simulink model "dog_test"  (R2015a)
settings: Solver=ode45  StartTime=0.0  StopTime=11796  RelTol=1e-3
InitFcn:
  | %% DSPBuilder Start
  | alt_dspbuilder_update_model(bdroot)
  | %% DSPBuilder End
libraries: allblocks_alteradspbuilder2 x539
(part 5 of 6)

== system dog_test/Gaussian_scale4/Subsystem ==
  valid_in : Inport
  eof_in : Inport  Port=2
  Comparator : allblocks_alteradspbuilder2/Comparator  direction=a == b  pipeline_display=0  allowFloatingPointOverride=on  logOutputs=off  logFile=C:\Users\ASUS\Desktop\sift_fpga_final\Gaussian filter 5x5\tb_dog_test\dog%5Ftest_Gaussian%5Fscale4_Subsystem_Comparator.fixedpointlog
  Comparator1 : allblocks_alteradspbuilder2/Comparator  direction=a < b  pipeline_display=0  allowFloatingPointOverride=on  logOutputs=off  logFile=C:\Users\ASUS\Desktop\sift_fpga_final\Gaussian filter 5x5\tb_dog_test\dog%5Ftest_Gaussian%5Fscale4_Subsystem_Comparator1.fixedpointlog
  Comparator2 : allblocks_alteradspbuilder2/Comparator  direction=a > b  pipeline_display=0  allowFloatingPointOverride=on  logOutputs=off  logFile=C:\Users\ASUS\Desktop\sift_fpga_final\Gaussian filter 5x5\tb_dog_test\dog%5Ftest_Gaussian%5Fscale4_Subsystem_Comparator2.fixedpointlog
  Comparator3 : allblocks_alteradspbuilder2/Comparator  direction=a > b  pipeline_display=0  allowFloatingPointOverride=on  logOutputs=off  logFile=C:\Users\ASUS\Desktop\sift_fpga_final\Gaussian filter 5x5\tb_dog_test\dog%5Ftest_Gaussian%5Fscale4_Subsystem_Comparator3.fixedpointlog
  Comparator4 : allblocks_alteradspbuilder2/Comparator  direction=a > b  pipeline_display=0  allowFloatingPointOverride=on  logOutputs=off  logFile=C:\Users\ASUS\Desktop\sift_fpga_final\Gaussian filter 5x5\tb_dog_test\dog%5Ftest_Gaussian%5Fscale4_Subsystem_Comparator4.fixedpointlog
  Comparator5 : allblocks_alteradspbuilder2/Comparator  direction=a > b  pipeline_display=0  allowFloatingPointOverride=on  logOutputs=off  logFile=C:\Users\ASUS\Desktop\sift_fpga_final\Gaussian filter 5x5\tb_dog_test\dog%5Ftest_Gaussian%5Fscale4_Subsystem_Comparator5.fixedpointlog
  Comparator6 : allblocks_alteradspbuilder2/Comparator  direction=a == b  pipeline_display=0  allowFloatingPointOverride=on  logOutputs=off  logFile=C:\Users\ASUS\Desktop\sift_fpga_final\Gaussian filter 5x5\tb_dog_test\dog%5Ftest_Gaussian%5Fscale4_Subsystem_Comparator6.fixedpointlog
  Comparator7 : allblocks_alteradspbuilder2/Comparator  direction=a == b  pipeline_display=0  allowFloatingPointOverride=on  logOutputs=off  logFile=C:\Users\ASUS\Desktop\sift_fpga_final\Gaussian filter 5x5\tb_dog_test\dog%5Ftest_Gaussian%5Fscale4_Subsystem_Comparator7.fixedpointlog
  Comparator8 : allblocks_alteradspbuilder2/Comparator  direction=a == b  pipeline_display=0  allowFloatingPointOverride=on  logOutputs=off  logFile=C:\Users\ASUS\Desktop\sift_fpga_final\Gaussian filter 5x5\tb_dog_test\dog%5Ftest_Gaussian%5Fscale4_Subsystem_Comparator8.fixedpointlog
  Constant : allblocks_alteradspbuilder2/Constant  mask_cst=643  BusType=Unsigned Integer  bwl=10  bwr=0  roundMode=Truncate  satMode=Wrap  SpecifyClock=off  allowFloatingPointOverride=on  logOutputs=off  logFile=C:\Users\ASUS\Desktop\sift_fpga_final\Gaussian filter 5x5\tb_dog_test\dog%5Ftest_Gaussian%5Fscale4_Subsystem_Constant.fixedpointlog
  Constant1 : allblocks_alteradspbuilder2/Constant  mask_cst=23  BusType=Unsigned Integer  bwl=10  bwr=0  roundMode=Truncate  satMode=Wrap  SpecifyClock=off  allowFloatingPointOverride=on  logOutputs=off  logFile=C:\Users\ASUS\Desktop\sift_fpga_final\Gaussian filter 5x5\tb_dog_test\dog%5Ftest_Gaussian%5Fscale4_Subsystem_Constant1.fixedpointlog
  Constant2 : allblocks_alteradspbuilder2/Constant  mask_cst=4  BusType=Unsigned Integer  bwl=10  bwr=0  roundMode=Truncate  satMode=Wrap  SpecifyClock=off  allowFloatingPointOverride=on  logOutputs=off  logFile=C:\Users\ASUS\Desktop\sift_fpga_final\Gaussian filter 5x5\tb_dog_test\dog%5Ftest_Gaussian%5Fscale4_Subsystem_Constant2.fixedpointlog
  Constant3 : allblocks_alteradspbuilder2/Constant  mask_cst=26  BusType=Unsigned Integer  bwl=10  bwr=0  roundMode=Truncate  satMode=Wrap  SpecifyClock=off  allowFloatingPointOverride=on  logOutputs=off  logFile=C:\Users\ASUS\Desktop\sift_fpga_final\Gaussian filter 5x5\tb_dog_test\dog%5Ftest_Gaussian%5Fscale4_Subsystem_Constant3.fixedpointlog
  Constant4 : allblocks_alteradspbuilder2/Constant  mask_cst=3  BusType=Unsigned Integer  bwl=10  bwr=0  roundMode=Truncate  satMode=Wrap  SpecifyClock=off  allowFloatingPointOverride=on  logOutputs=off  logFile=C:\Users\ASUS\Desktop\sift_fpga_final\Gaussian filter 5x5\tb_dog_test\dog%5Ftest_Gaussian%5Fscale4_Subsystem_Constant4.fixedpointlog
  Constant5 : allblocks_alteradspbuilder2/Constant  mask_cst=0  BusType=Unsigned Integer  bwl=10  bwr=0  roundMode=Truncate  satMode=Wrap  SpecifyClock=off  allowFloatingPointOverride=on  logOutputs=off  logFile=C:\Users\ASUS\Desktop\sift_fpga_final\Gaussian filter 5x5\tb_dog_test\dog%5Ftest_Gaussian%5Fscale4_Subsystem_Constant5.fixedpointlog
  Constant6 : allblocks_alteradspbuilder2/Constant  mask_cst=23  BusType=Unsigned Integer  bwl=10  bwr=0  roundMode=Truncate  satMode=Wrap  SpecifyClock=off  allowFloatingPointOverride=on  logOutputs=off  logFile=C:\Users\ASUS\Desktop\sift_fpga_final\Gaussian filter 5x5\tb_dog_test\dog%5Ftest_Gaussian%5Fscale4_Subsystem_Constant6.fixedpointlog
  Constant7 : allblocks_alteradspbuilder2/Constant  mask_cst=4  BusType=Unsigned Integer  bwl=10  bwr=0  roundMode=Truncate  satMode=Wrap  SpecifyClock=off  allowFloatingPointOverride=on  logOutputs=off  logFile=C:\Users\ASUS\Desktop\sift_fpga_final\Gaussian filter 5x5\tb_dog_test\dog%5Ftest_Gaussian%5Fscale4_Subsystem_Constant7.fixedpointlog
  Constant8 : allblocks_alteradspbuilder2/Constant  mask_cst=27  BusType=Unsigned Integer  bwl=10  bwr=0  roundMode=Truncate  satMode=Wrap  SpecifyClock=off  allowFloatingPointOverride=on  logOutputs=off  logFile=C:\Users\ASUS\Desktop\sift_fpga_final\Gaussian filter 5x5\tb_dog_test\dog%5Ftest_Gaussian%5Fscale4_Subsystem_Constant8.fixedpointlog
  Counter : allblocks_alteradspbuilder2/Counter  BusType=Unsigned Integer  bwl=10  bwr=0  use_modulo=on  modulo=644  SpecifyClock=off  direction=Increment  use_sload=off  use_sset=off  svalue=1  use_clk_ena=off  use_ena=on  use_sclr=on  pipeline_display=1
  Counter1 : allblocks_alteradspbuilder2/Counter  BusType=Unsigned Integer  bwl=10  bwr=0  use_modulo=on  modulo=484  SpecifyClock=off  direction=Increment  use_sload=off  use_sset=off  svalue=1  use_clk_ena=off  use_ena=on  use_sclr=on  pipeline_display=1
  Counter2 : allblocks_alteradspbuilder2/Counter  BusType=Unsigned Integer  bwl=5  bwr=0  use_modulo=on  modulo=24  SpecifyClock=off  direction=Increment  use_sload=off  use_sset=on  svalue=1  use_clk_ena=off  use_ena=on  use_sclr=off  pipeline_display=1
  Logical Bit Operator{,1..3,5..6} (6 alike) : allblocks_alteradspbuilder2/Logical Bit Operator  LogicalOperator=AND  user_inputs=2  pipeline_display=0
  Logical Bit Operator4 : allblocks_alteradspbuilder2/Logical Bit Operator  LogicalOperator=OR  user_inputs=3  pipeline_display=0
  Logical Bit Operator7 : allblocks_alteradspbuilder2/Logical Bit Operator  LogicalOperator=AND  user_inputs=3  pipeline_display=0
  valid_out : Outport
  sof_out : Outport  Port=2
  eof_out : Outport  Port=3
  wires:
  Logical Bit Operator3/1 -> Logical Bit Operator4/2
  Counter2/1 -> [counter_eof]
  [valid_in] -> Logical Bit Operator1/1
  Constant1/1 -> Comparator1/2
  Constant2/1 -> Comparator2/2
  Constant3/1 -> Comparator3/2
  Logical Bit Operator4/1 -> Logical Bit Operator1/2
  [valid_in] -> Logical Bit Operator5/1
  Comparator/1 -> Logical Bit Operator/2
  [counter_col] -> Comparator3/1
  [counter_eof] -> Comparator5/1
  [counter_col] -> Comparator/1
  Constant5/1 -> Comparator5/2
  eof_in/1 -> [eof_in]
  [eof_in] -> Counter1/2
  Logical Bit Operator1/1 -> [valid_out]
  Constant/1 -> Comparator/2
  Logical Bit Operator/1 -> Counter1/1
  Comparator2/1 -> Logical Bit Operator2/2
  Comparator3/1 -> Logical Bit Operator3/1
  Comparator4/1 -> Logical Bit Operator3/2
  Logical Bit Operator2/1 -> Logical Bit Operator4/1
  valid_in/1 -> [valid_in]
  [eof_in] -> Counter/2
  Counter1/1 -> [counter_row]
  [counter_row] -> Comparator2/1
  [counter_row] -> Comparator4/1
  Constant4/1 -> Comparator4/2
  [valid_in] -> Logical Bit Operator/1, Counter/1
  Counter/1 -> [counter_col]
  [counter_col] -> Comparator1/1
  Comparator1/1 -> Logical Bit Operator2/1
  Comparator7/1 -> Logical Bit Operator7/2
  [valid_in] -> Logical Bit Operator7/1
  Constant6/1 -> Comparator6/2
  [sof_out] -> sof_out/1
  [counter_row] -> Comparator7/1
  Comparator8/1 -> Logical Bit Operator7/3
  [counter_col] -> Comparator8/1
  [valid_in] -> Logical Bit Operator6/1
  [eof_out] -> eof_out/1
  Logical Bit Operator7/1 -> [sof_out]
  [valid_out] -> valid_out/1
  [counter_eof] -> Comparator6/1
  Constant8/1 -> Comparator8/2
  Comparator6/1 -> Logical Bit Operator6/2
  Comparator5/1 -> Logical Bit Operator5/2, Logical Bit Operator4/3
  Logical Bit Operator6/1 -> [eof_out]
  Constant7/1 -> Comparator7/2
  [eof_in] -> Counter2/1
  Logical Bit Operator5/1 -> Counter2/2

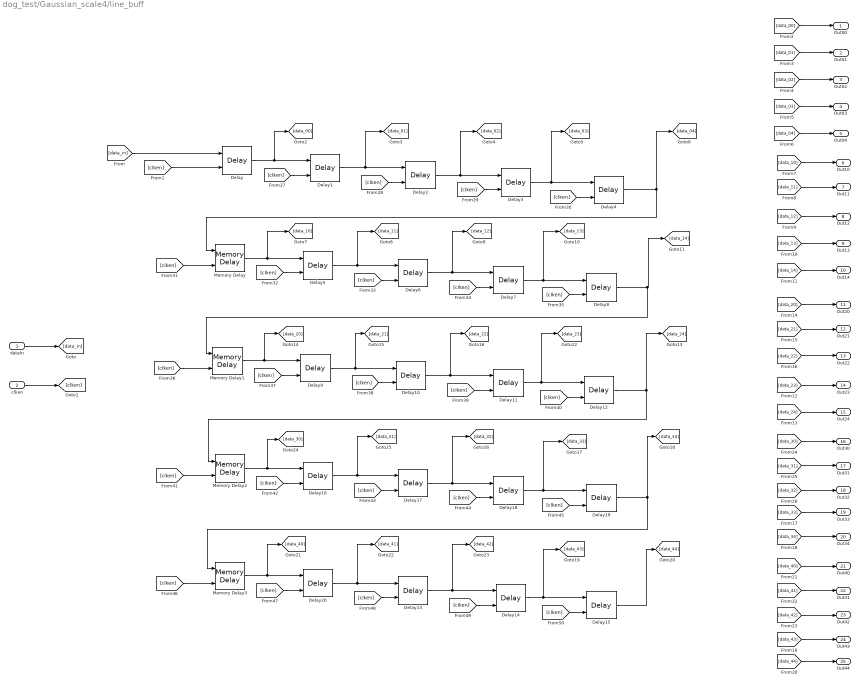
== system dog_test/Gaussian_scale4/line_buff ==
  dataIn : Inport
  clken : Inport  Port=2
  Delay : allblocks_alteradspbuilder2/Delay  pipeline=1  pipeline_display=1  ClockPhase=1  use_ena=on  use_sclr=off  allowFloatingPointOverride=on  logOutputs=off  logFile=C:\Users\ASUS\Desktop\sift_fpga_final\Gaussian filter 5x5\tb_dog_test\dog%5Ftest_Gaussian%5Fscale4_line%5Fbuff_Delay.fixedpointlog  use_init=off  reset_value=1
  Delay1 : allblocks_alteradspbuilder2/Delay  pipeline=1  pipeline_display=1  ClockPhase=1  use_ena=on  use_sclr=off  allowFloatingPointOverride=on  logOutputs=off  logFile=C:\Users\ASUS\Desktop\sift_fpga_final\Gaussian filter 5x5\tb_dog_test\dog%5Ftest_Gaussian%5Fscale4_line%5Fbuff_Delay1.fixedpointlog  use_init=off  reset_value=1
  Delay10 : allblocks_alteradspbuilder2/Delay  pipeline=1  pipeline_display=1  ClockPhase=1  use_ena=on  use_sclr=off  allowFloatingPointOverride=on  logOutputs=off  logFile=C:\Users\ASUS\Desktop\sift_fpga_final\Gaussian filter 5x5\tb_dog_test\dog%5Ftest_Gaussian%5Fscale4_line%5Fbuff_Delay10.fixedpointlog  use_init=off  reset_value=1
  Delay11 : allblocks_alteradspbuilder2/Delay  pipeline=1  pipeline_display=1  ClockPhase=1  use_ena=on  use_sclr=off  allowFloatingPointOverride=on  logOutputs=off  logFile=C:\Users\ASUS\Desktop\sift_fpga_final\Gaussian filter 5x5\tb_dog_test\dog%5Ftest_Gaussian%5Fscale4_line%5Fbuff_Delay11.fixedpointlog  use_init=off  reset_value=1
  Delay12 : allblocks_alteradspbuilder2/Delay  pipeline=1  pipeline_display=1  ClockPhase=1  use_ena=on  use_sclr=off  allowFloatingPointOverride=on  logOutputs=off  logFile=C:\Users\ASUS\Desktop\sift_fpga_final\Gaussian filter 5x5\tb_dog_test\dog%5Ftest_Gaussian%5Fscale4_line%5Fbuff_Delay12.fixedpointlog  use_init=off  reset_value=1
  Delay13 : allblocks_alteradspbuilder2/Delay  pipeline=1  pipeline_display=1  ClockPhase=1  use_ena=on  use_sclr=off  allowFloatingPointOverride=on  logOutputs=off  logFile=C:\Users\ASUS\Desktop\sift_fpga_final\Gaussian filter 5x5\tb_dog_test\dog%5Ftest_Gaussian%5Fscale4_line%5Fbuff_Delay13.fixedpointlog  use_init=off  reset_value=1
  Delay14 : allblocks_alteradspbuilder2/Delay  pipeline=1  pipeline_display=1  ClockPhase=1  use_ena=on  use_sclr=off  allowFloatingPointOverride=on  logOutputs=off  logFile=C:\Users\ASUS\Desktop\sift_fpga_final\Gaussian filter 5x5\tb_dog_test\dog%5Ftest_Gaussian%5Fscale4_line%5Fbuff_Delay14.fixedpointlog  use_init=off  reset_value=1
  Delay15 : allblocks_alteradspbuilder2/Delay  pipeline=1  pipeline_display=1  ClockPhase=1  use_ena=on  use_sclr=off  allowFloatingPointOverride=on  logOutputs=off  logFile=C:\Users\ASUS\Desktop\sift_fpga_final\Gaussian filter 5x5\tb_dog_test\dog%5Ftest_Gaussian%5Fscale4_line%5Fbuff_Delay15.fixedpointlog  use_init=off  reset_value=1
  Delay16 : allblocks_alteradspbuilder2/Delay  pipeline=1  pipeline_display=1  ClockPhase=1  use_ena=on  use_sclr=off  allowFloatingPointOverride=on  logOutputs=off  logFile=C:\Users\ASUS\Desktop\sift_fpga_final\Gaussian filter 5x5\tb_dog_test\dog%5Ftest_Gaussian%5Fscale4_line%5Fbuff_Delay16.fixedpointlog  use_init=off  reset_value=1
  Delay17 : allblocks_alteradspbuilder2/Delay  pipeline=1  pipeline_display=1  ClockPhase=1  use_ena=on  use_sclr=off  allowFloatingPointOverride=on  logOutputs=off  logFile=C:\Users\ASUS\Desktop\sift_fpga_final\Gaussian filter 5x5\tb_dog_test\dog%5Ftest_Gaussian%5Fscale4_line%5Fbuff_Delay17.fixedpointlog  use_init=off  reset_value=1
  Delay18 : allblocks_alteradspbuilder2/Delay  pipeline=1  pipeline_display=1  ClockPhase=1  use_ena=on  use_sclr=off  allowFloatingPointOverride=on  logOutputs=off  logFile=C:\Users\ASUS\Desktop\sift_fpga_final\Gaussian filter 5x5\tb_dog_test\dog%5Ftest_Gaussian%5Fscale4_line%5Fbuff_Delay18.fixedpointlog  use_init=off  reset_value=1
  Delay19 : allblocks_alteradspbuilder2/Delay  pipeline=1  pipeline_display=1  ClockPhase=1  use_ena=on  use_sclr=off  allowFloatingPointOverride=on  logOutputs=off  logFile=C:\Users\ASUS\Desktop\sift_fpga_final\Gaussian filter 5x5\tb_dog_test\dog%5Ftest_Gaussian%5Fscale4_line%5Fbuff_Delay19.fixedpointlog  use_init=off  reset_value=1
  Delay2 : allblocks_alteradspbuilder2/Delay  pipeline=1  pipeline_display=1  ClockPhase=1  use_ena=on  use_sclr=off  allowFloatingPointOverride=on  logOutputs=off  logFile=C:\Users\ASUS\Desktop\sift_fpga_final\Gaussian filter 5x5\tb_dog_test\dog%5Ftest_Gaussian%5Fscale4_line%5Fbuff_Delay2.fixedpointlog  use_init=off  reset_value=1
  Delay20 : allblocks_alteradspbuilder2/Delay  pipeline=1  pipeline_display=1  ClockPhase=1  use_ena=on  use_sclr=off  allowFloatingPointOverride=on  logOutputs=off  logFile=C:\Users\ASUS\Desktop\sift_fpga_final\Gaussian filter 5x5\tb_dog_test\dog%5Ftest_Gaussian%5Fscale4_line%5Fbuff_Delay20.fixedpointlog  use_init=off  reset_value=1
  Delay3 : allblocks_alteradspbuilder2/Delay  pipeline=1  pipeline_display=1  ClockPhase=1  use_ena=on  use_sclr=off  allowFloatingPointOverride=on  logOutputs=off  logFile=C:\Users\ASUS\Desktop\sift_fpga_final\Gaussian filter 5x5\tb_dog_test\dog%5Ftest_Gaussian%5Fscale4_line%5Fbuff_Delay3.fixedpointlog  use_init=off  reset_value=1
  Delay4 : allblocks_alteradspbuilder2/Delay  pipeline=1  pipeline_display=1  ClockPhase=1  use_ena=on  use_sclr=off  allowFloatingPointOverride=on  logOutputs=off  logFile=C:\Users\ASUS\Desktop\sift_fpga_final\Gaussian filter 5x5\tb_dog_test\dog%5Ftest_Gaussian%5Fscale4_line%5Fbuff_Delay4.fixedpointlog  use_init=off  reset_value=1
  Delay5 : allblocks_alteradspbuilder2/Delay  pipeline=1  pipeline_display=1  ClockPhase=1  use_ena=on  use_sclr=off  allowFloatingPointOverride=on  logOutputs=off  logFile=C:\Users\ASUS\Desktop\sift_fpga_final\Gaussian filter 5x5\tb_dog_test\dog%5Ftest_Gaussian%5Fscale4_line%5Fbuff_Delay5.fixedpointlog  use_init=off  reset_value=1
  Delay6 : allblocks_alteradspbuilder2/Delay  pipeline=1  pipeline_display=1  ClockPhase=1  use_ena=on  use_sclr=off  allowFloatingPointOverride=on  logOutputs=off  logFile=C:\Users\ASUS\Desktop\sift_fpga_final\Gaussian filter 5x5\tb_dog_test\dog%5Ftest_Gaussian%5Fscale4_line%5Fbuff_Delay6.fixedpointlog  use_init=off  reset_value=1
  Delay7 : allblocks_alteradspbuilder2/Delay  pipeline=1  pipeline_display=1  ClockPhase=1  use_ena=on  use_sclr=off  allowFloatingPointOverride=on  logOutputs=off  logFile=C:\Users\ASUS\Desktop\sift_fpga_final\Gaussian filter 5x5\tb_dog_test\dog%5Ftest_Gaussian%5Fscale4_line%5Fbuff_Delay7.fixedpointlog  use_init=off  reset_value=1
  Delay8 : allblocks_alteradspbuilder2/Delay  pipeline=1  pipeline_display=1  ClockPhase=1  use_ena=on  use_sclr=off  allowFloatingPointOverride=on  logOutputs=off  logFile=C:\Users\ASUS\Desktop\sift_fpga_final\Gaussian filter 5x5\tb_dog_test\dog%5Ftest_Gaussian%5Fscale4_line%5Fbuff_Delay8.fixedpointlog  use_init=off  reset_value=1
  Delay9 : allblocks_alteradspbuilder2/Delay  pipeline=1  pipeline_display=1  ClockPhase=1  use_ena=on  use_sclr=off  allowFloatingPointOverride=on  logOutputs=off  logFile=C:\Users\ASUS\Desktop\sift_fpga_final\Gaussian filter 5x5\tb_dog_test\dog%5Ftest_Gaussian%5Fscale4_line%5Fbuff_Delay9.fixedpointlog  use_init=off  reset_value=1
  Memory Delay : allblocks_alteradspbuilder2/Memory Delay  BusType=Unsigned Integer  bwl=8  bwr=0  pipeline=640  pipeline_display=640  ram_type=AUTO  use_ena=on  use_sclr=off  allowFloatingPointOverride=on  logOutputs=off  logFile=C:\Users\ASUS\Desktop\sift_fpga_final\Gaussian filter 5x5\tb_dog_test\dog%5Ftest_Gaussian%5Fscale4_line%5Fbuff_Memory+Delay.fixedpointlog
  Memory Delay1 : allblocks_alteradspbuilder2/Memory Delay  BusType=Unsigned Integer  bwl=8  bwr=0  pipeline=640  pipeline_display=640  ram_type=AUTO  use_ena=on  use_sclr=off  allowFloatingPointOverride=on  logOutputs=off  logFile=C:\Users\ASUS\Desktop\sift_fpga_final\Gaussian filter 5x5\tb_dog_test\dog%5Ftest_Gaussian%5Fscale4_line%5Fbuff_Memory+Delay1.fixedpointlog
  Memory Delay2 : allblocks_alteradspbuilder2/Memory Delay  BusType=Unsigned Integer  bwl=8  bwr=0  pipeline=640  pipeline_display=640  ram_type=AUTO  use_ena=on  use_sclr=off  allowFloatingPointOverride=on  logOutputs=off  logFile=C:\Users\ASUS\Desktop\sift_fpga_final\Gaussian filter 5x5\tb_dog_test\dog%5Ftest_Gaussian%5Fscale4_line%5Fbuff_Memory+Delay2.fixedpointlog
  Memory Delay3 : allblocks_alteradspbuilder2/Memory Delay  BusType=Unsigned Integer  bwl=8  bwr=0  pipeline=640  pipeline_display=640  ram_type=AUTO  use_ena=on  use_sclr=off  allowFloatingPointOverride=on  logOutputs=off  logFile=C:\Users\ASUS\Desktop\sift_fpga_final\Gaussian filter 5x5\tb_dog_test\dog%5Ftest_Gaussian%5Fscale4_line%5Fbuff_Memory+Delay3.fixedpointlog
  Out00 : Outport
  Out01 : Outport  Port=2
  Out02 : Outport  Port=3
  Out03 : Outport  Port=4
  Out04 : Outport  Port=5
  Out10 : Outport  Port=6
  Out11 : Outport  Port=7
  Out12 : Outport  Port=8
  Out13 : Outport  Port=9
  Out14 : Outport  Port=10
  Out20 : Outport  Port=11
  Out21 : Outport  Port=12
  Out22 : Outport  Port=13
  Out23 : Outport  Port=14
  Out24 : Outport  Port=15
  Out30 : Outport  Port=16
  Out31 : Outport  Port=17
  Out32 : Outport  Port=18
  Out33 : Outport  Port=19
  Out34 : Outport  Port=20
  Out40 : Outport  Port=21
  Out41 : Outport  Port=22
  Out42 : Outport  Port=23
  Out43 : Outport  Port=24
  Out44 : Outport  Port=25
  wires:
  [clken] -> Delay9/2
  [data_04] -> Out04/1
  [data_02] -> Out02/1
  [clken] -> Memory Delay1/2
  [data_44] -> Out44/1
  [data_33] -> Out33/1
  [clken] -> Delay4/2
  [clken] -> Delay11/2
  [data_32] -> Out32/1
  [data_31] -> Out31/1
  [data_40] -> Out40/1
  [data_43] -> Out43/1
  [data_42] -> Out42/1
  Delay11/1 -> [data_23], Delay12/1
  Memory Delay1/1 -> [data_20], Delay9/1
  [data_41] -> Out41/1
  Delay9/1 -> [data_21], Delay10/1
  [clken] -> Delay12/2
  [data_34] -> Out34/1
  [data_30] -> Out30/1
  Delay/1 -> [data_00], Delay1/1
  [clken] -> Delay1/2
  [clken] -> Delay/2
  [data_03] -> Out03/1
  [clken] -> Delay10/2
  Delay8/1 -> Memory Delay1/1, [data_14]
  Delay10/1 -> [data_22], Delay11/1
  [data_12] -> Out12/1
  dataIn/1 -> [data_in]
  Memory Delay3/1 -> [data_40], Delay20/1
  [clken] -> Memory Delay/2
  [clken] -> Delay2/2
  [data_22] -> Out22/1
  [clken] -> Delay14/2
  Delay17/1 -> [data_32], Delay18/1
  [clken] -> Delay20/2
  [data_10] -> Out10/1
  [data_21] -> Out21/1
  Delay12/1 -> [data_24], Memory Delay2/1
  Delay4/1 -> Memory Delay/1, [data_04]
  [clken] -> Delay3/2
  Delay2/1 -> [data_02], Delay3/1
  [clken] -> Memory Delay2/2
  [data_23] -> Out23/1
  [data_13] -> Out13/1
  clken/1 -> [clken]
  [data_11] -> Out11/1
  Delay18/1 -> [data_33], Delay19/1
  [data_20] -> Out20/1
  Delay1/1 -> [data_01], Delay2/1
  [data_24] -> Out24/1
  Memory Delay2/1 -> [data_30], Delay16/1
  [clken] -> Delay16/2
  [data_14] -> Out14/1
  [data_00] -> Out00/1
  [clken] -> Delay15/2
  [clken] -> Memory Delay3/2
  [data_01] -> Out01/1
  [data_in] -> Delay/1
  [clken] -> Delay7/2
  Delay19/1 -> Memory Delay3/1, [data_34]
  Delay14/1 -> [data_43], Delay15/1
  Memory Delay/1 -> [data_10], Delay5/1
  Delay5/1 -> [data_11], Delay6/1
  Delay16/1 -> [data_31], Delay17/1
  [clken] -> Delay6/2
  Delay6/1 -> [data_12], Delay7/1
  [clken] -> Delay13/2
  Delay3/1 -> [data_03], Delay4/1
  Delay15/1 -> [data_44]
  [clken] -> Delay18/2
  Delay13/1 -> [data_42], Delay14/1
  [clken] -> Delay5/2
  Delay7/1 -> [data_13], Delay8/1
  Delay20/1 -> [data_41], Delay13/1
  [clken] -> Delay17/2
  [clken] -> Delay19/2
  [clken] -> Delay8/2

== system dog_test/calculate_key_point/Subsystem ==
  dataIn : Inport
  clken : Inport  Port=2
  Delay : allblocks_alteradspbuilder2/Delay  pipeline=1  pipeline_display=1  ClockPhase=1  use_ena=on  use_sclr=off  allowFloatingPointOverride=on  logOutputs=off  logFile=C:\Users\ASUS\Desktop\sift_fpga_final\Gaussian filter 5x5\tb_dog_test\dog%5Ftest_calculate%5Fkey%5Fpoint_Subsystem_Delay.fixedpointlog  use_init=off  reset_value=1
  Delay1 : allblocks_alteradspbuilder2/Delay  pipeline=1  pipeline_display=1  ClockPhase=1  use_ena=on  use_sclr=off  allowFloatingPointOverride=on  logOutputs=off  logFile=C:\Users\ASUS\Desktop\sift_fpga_final\Gaussian filter 5x5\tb_dog_test\dog%5Ftest_calculate%5Fkey%5Fpoint_Subsystem_Delay1.fixedpointlog  use_init=off  reset_value=1
  Delay10 : allblocks_alteradspbuilder2/Delay  pipeline=1  pipeline_display=1  ClockPhase=1  use_ena=on  use_sclr=off  allowFloatingPointOverride=on  logOutputs=off  logFile=C:\Users\ASUS\Desktop\sift_fpga_final\Gaussian filter 5x5\tb_dog_test\dog%5Ftest_calculate%5Fkey%5Fpoint_Subsystem_Delay10.fixedpointlog  use_init=off  reset_value=1
  Delay2 : allblocks_alteradspbuilder2/Delay  pipeline=1  pipeline_display=1  ClockPhase=1  use_ena=on  use_sclr=off  allowFloatingPointOverride=on  logOutputs=off  logFile=C:\Users\ASUS\Desktop\sift_fpga_final\Gaussian filter 5x5\tb_dog_test\dog%5Ftest_calculate%5Fkey%5Fpoint_Subsystem_Delay2.fixedpointlog  use_init=off  reset_value=1
  Delay5 : allblocks_alteradspbuilder2/Delay  pipeline=1  pipeline_display=1  ClockPhase=1  use_ena=on  use_sclr=off  allowFloatingPointOverride=on  logOutputs=off  logFile=C:\Users\ASUS\Desktop\sift_fpga_final\Gaussian filter 5x5\tb_dog_test\dog%5Ftest_calculate%5Fkey%5Fpoint_Subsystem_Delay5.fixedpointlog  use_init=off  reset_value=1
  Delay6 : allblocks_alteradspbuilder2/Delay  pipeline=1  pipeline_display=1  ClockPhase=1  use_ena=on  use_sclr=off  allowFloatingPointOverride=on  logOutputs=off  logFile=C:\Users\ASUS\Desktop\sift_fpga_final\Gaussian filter 5x5\tb_dog_test\dog%5Ftest_calculate%5Fkey%5Fpoint_Subsystem_Delay6.fixedpointlog  use_init=off  reset_value=1
  Delay9 : allblocks_alteradspbuilder2/Delay  pipeline=1  pipeline_display=1  ClockPhase=1  use_ena=on  use_sclr=off  allowFloatingPointOverride=on  logOutputs=off  logFile=C:\Users\ASUS\Desktop\sift_fpga_final\Gaussian filter 5x5\tb_dog_test\dog%5Ftest_calculate%5Fkey%5Fpoint_Subsystem_Delay9.fixedpointlog  use_init=off  reset_value=1
  Memory Delay : allblocks_alteradspbuilder2/Memory Delay  BusType=Unsigned Integer  bwl=8  bwr=0  pipeline=638  pipeline_display=638  ram_type=AUTO  use_ena=on  use_sclr=off  allowFloatingPointOverride=on  logOutputs=off  logFile=C:\Users\ASUS\Desktop\sift_fpga_final\Gaussian filter 5x5\tb_dog_test\dog%5Ftest_calculate%5Fkey%5Fpoint_Subsystem_Memory+Delay.fixedpointlog
  Memory Delay1 : allblocks_alteradspbuilder2/Memory Delay  BusType=Unsigned Integer  bwl=8  bwr=0  pipeline=638  pipeline_display=638  ram_type=AUTO  use_ena=on  use_sclr=off  allowFloatingPointOverride=on  logOutputs=off  logFile=C:\dog%5Ftest_calculate%5Fkey%5Fpoint_Subsystem_Memory+Delay1.fixedpointlog
  Out00 : Outport
  Out01 : Outport  Port=2
  Out02 : Outport  Port=3
  Out10 : Outport  Port=4
  Out11 : Outport  Port=5
  Out12 : Outport  Port=6
  Out20 : Outport  Port=7
  Out21 : Outport  Port=8
  Out22 : Outport  Port=9
  wires:
  Delay1/1 -> [data_01], Delay2/1
  Delay/1 -> [data_00], Delay1/1
  Delay9/1 -> [data_21], Delay10/1
  [clken] -> Delay10/2
  [clken] -> Memory Delay1/2
  Delay6/1 -> Memory Delay1/1, [data_12]
  Memory Delay1/1 -> [data_20], Delay9/1
  [clken] -> Delay9/2
  [data_02] -> Out02/1
  [clken] -> Delay1/2
  [clken] -> Delay/2
  [data_in] -> Delay/1
  [clken] -> Delay2/2
  Delay2/1 -> Memory Delay/1, [data_02]
  [data_22] -> Out22/1
  Delay10/1 -> [data_22]
  clken/1 -> [clken]
  [data_21] -> Out21/1
  [data_20] -> Out20/1
  [data_10] -> Out10/1
  Memory Delay/1 -> [data_10], Delay5/1
  [clken] -> Memory Delay/2
  [clken] -> Delay6/2
  Delay5/1 -> [data_11], Delay6/1
  [data_12] -> Out12/1
  [data_00] -> Out00/1
  [data_01] -> Out01/1
  [clken] -> Delay5/2
  [data_11] -> Out11/1
  dataIn/1 -> [data_in]

== system dog_test/calculate_key_point/Subsystem1 ==
  dataIn : Inport
  clken : Inport  Port=2
  Delay : allblocks_alteradspbuilder2/Delay  pipeline=1  pipeline_display=1  ClockPhase=1  use_ena=on  use_sclr=off  allowFloatingPointOverride=on  logOutputs=off  logFile=C:\Users\ASUS\Desktop\sift_fpga_final\Gaussian filter 5x5\tb_dog_test\dog%5Ftest_calculate%5Fkey%5Fpoint_Subsystem1_Delay.fixedpointlog  use_init=off  reset_value=1
  Delay1 : allblocks_alteradspbuilder2/Delay  pipeline=1  pipeline_display=1  ClockPhase=1  use_ena=on  use_sclr=off  allowFloatingPointOverride=on  logOutputs=off  logFile=C:\Users\ASUS\Desktop\sift_fpga_final\Gaussian filter 5x5\tb_dog_test\dog%5Ftest_calculate%5Fkey%5Fpoint_Subsystem1_Delay1.fixedpointlog  use_init=off  reset_value=1
  Delay10 : allblocks_alteradspbuilder2/Delay  pipeline=1  pipeline_display=1  ClockPhase=1  use_ena=on  use_sclr=off  allowFloatingPointOverride=on  logOutputs=off  logFile=C:\Users\ASUS\Desktop\sift_fpga_final\Gaussian filter 5x5\tb_dog_test\dog%5Ftest_calculate%5Fkey%5Fpoint_Subsystem1_Delay10.fixedpointlog  use_init=off  reset_value=1
  Delay2 : allblocks_alteradspbuilder2/Delay  pipeline=1  pipeline_display=1  ClockPhase=1  use_ena=on  use_sclr=off  allowFloatingPointOverride=on  logOutputs=off  logFile=C:\Users\ASUS\Desktop\sift_fpga_final\Gaussian filter 5x5\tb_dog_test\dog%5Ftest_calculate%5Fkey%5Fpoint_Subsystem1_Delay2.fixedpointlog  use_init=off  reset_value=1
  Delay5 : allblocks_alteradspbuilder2/Delay  pipeline=1  pipeline_display=1  ClockPhase=1  use_ena=on  use_sclr=off  allowFloatingPointOverride=on  logOutputs=off  logFile=C:\Users\ASUS\Desktop\sift_fpga_final\Gaussian filter 5x5\tb_dog_test\dog%5Ftest_calculate%5Fkey%5Fpoint_Subsystem1_Delay5.fixedpointlog  use_init=off  reset_value=1
  Delay6 : allblocks_alteradspbuilder2/Delay  pipeline=1  pipeline_display=1  ClockPhase=1  use_ena=on  use_sclr=off  allowFloatingPointOverride=on  logOutputs=off  logFile=C:\Users\ASUS\Desktop\sift_fpga_final\Gaussian filter 5x5\tb_dog_test\dog%5Ftest_calculate%5Fkey%5Fpoint_Subsystem1_Delay6.fixedpointlog  use_init=off  reset_value=1
  Delay9 : allblocks_alteradspbuilder2/Delay  pipeline=1  pipeline_display=1  ClockPhase=1  use_ena=on  use_sclr=off  allowFloatingPointOverride=on  logOutputs=off  logFile=C:\Users\ASUS\Desktop\sift_fpga_final\Gaussian filter 5x5\tb_dog_test\dog%5Ftest_calculate%5Fkey%5Fpoint_Subsystem1_Delay9.fixedpointlog  use_init=off  reset_value=1
  Memory Delay : allblocks_alteradspbuilder2/Memory Delay  BusType=Unsigned Integer  bwl=8  bwr=0  pipeline=638  pipeline_display=638  ram_type=AUTO  use_ena=on  use_sclr=off  allowFloatingPointOverride=on  logOutputs=off  logFile=C:\Users\ASUS\Desktop\sift_fpga_final\Gaussian filter 5x5\tb_dog_test\dog%5Ftest_calculate%5Fkey%5Fpoint_Subsystem1_Memory+Delay.fixedpointlog
  Memory Delay1 : allblocks_alteradspbuilder2/Memory Delay  BusType=Unsigned Integer  bwl=8  bwr=0  pipeline=638  pipeline_display=638  ram_type=AUTO  use_ena=on  use_sclr=off  allowFloatingPointOverride=on  logOutputs=off  logFile=C:\Users\ASUS\Desktop\sift_fpga_final\Gaussian filter 5x5\tb_dog_test\dog%5Ftest_calculate%5Fkey%5Fpoint_Subsystem1_Memory+Delay1.fixedpointlog
  Out00 : Outport
  Out01 : Outport  Port=2
  Out02 : Outport  Port=3
  Out10 : Outport  Port=4
  Out11 : Outport  Port=5
  Out12 : Outport  Port=6
  Out20 : Outport  Port=7
  Out21 : Outport  Port=8
  Out22 : Outport  Port=9
  wires:
  Delay1/1 -> [data_01], Delay2/1
  Delay/1 -> [data_00], Delay1/1
  Delay9/1 -> [data_21], Delay10/1
  [clken] -> Delay10/2
  [clken] -> Memory Delay1/2
  Delay6/1 -> Memory Delay1/1, [data_12]
  Memory Delay1/1 -> [data_20], Delay9/1
  [clken] -> Delay9/2
  [data_02] -> Out02/1
  [clken] -> Delay1/2
  [clken] -> Delay/2
  [data_in] -> Delay/1
  [clken] -> Delay2/2
  Delay2/1 -> Memory Delay/1, [data_02]
  [data_22] -> Out22/1
  Delay10/1 -> [data_22]
  clken/1 -> [clken]
  [data_21] -> Out21/1
  [data_20] -> Out20/1
  [data_10] -> Out10/1
  Memory Delay/1 -> [data_10], Delay5/1
  [clken] -> Memory Delay/2
  [clken] -> Delay6/2
  Delay5/1 -> [data_11], Delay6/1
  [data_12] -> Out12/1
  [data_00] -> Out00/1
  [data_01] -> Out01/1
  [clken] -> Delay5/2
  [data_11] -> Out11/1
  dataIn/1 -> [data_in]

== system dog_test/calculate_key_point/Subsystem2 ==
  dataIn : Inport
  clken : Inport  Port=2
  Delay : allblocks_alteradspbuilder2/Delay  pipeline=1  pipeline_display=1  ClockPhase=1  use_ena=on  use_sclr=off  allowFloatingPointOverride=on  logOutputs=off  logFile=C:\Users\ASUS\Desktop\sift_fpga_final\Gaussian filter 5x5\tb_dog_test\dog%5Ftest_calculate%5Fkey%5Fpoint_Subsystem2_Delay.fixedpointlog  use_init=off  reset_value=1
  Delay1 : allblocks_alteradspbuilder2/Delay  pipeline=1  pipeline_display=1  ClockPhase=1  use_ena=on  use_sclr=off  allowFloatingPointOverride=on  logOutputs=off  logFile=C:\Users\ASUS\Desktop\sift_fpga_final\Gaussian filter 5x5\tb_dog_test\dog%5Ftest_calculate%5Fkey%5Fpoint_Subsystem2_Delay1.fixedpointlog  use_init=off  reset_value=1
  Delay10 : allblocks_alteradspbuilder2/Delay  pipeline=1  pipeline_display=1  ClockPhase=1  use_ena=on  use_sclr=off  allowFloatingPointOverride=on  logOutputs=off  logFile=C:\Users\ASUS\Desktop\sift_fpga_final\Gaussian filter 5x5\tb_dog_test\dog%5Ftest_calculate%5Fkey%5Fpoint_Subsystem2_Delay10.fixedpointlog  use_init=off  reset_value=1
  Delay2 : allblocks_alteradspbuilder2/Delay  pipeline=1  pipeline_display=1  ClockPhase=1  use_ena=on  use_sclr=off  allowFloatingPointOverride=on  logOutputs=off  logFile=C:\Users\ASUS\Desktop\sift_fpga_final\Gaussian filter 5x5\tb_dog_test\dog%5Ftest_calculate%5Fkey%5Fpoint_Subsystem2_Delay2.fixedpointlog  use_init=off  reset_value=1
  Delay5 : allblocks_alteradspbuilder2/Delay  pipeline=1  pipeline_display=1  ClockPhase=1  use_ena=on  use_sclr=off  allowFloatingPointOverride=on  logOutputs=off  logFile=C:\Users\ASUS\Desktop\sift_fpga_final\Gaussian filter 5x5\tb_dog_test\dog%5Ftest_calculate%5Fkey%5Fpoint_Subsystem2_Delay5.fixedpointlog  use_init=off  reset_value=1
  Delay6 : allblocks_alteradspbuilder2/Delay  pipeline=1  pipeline_display=1  ClockPhase=1  use_ena=on  use_sclr=off  allowFloatingPointOverride=on  logOutputs=off  logFile=C:\Users\ASUS\Desktop\sift_fpga_final\Gaussian filter 5x5\tb_dog_test\dog%5Ftest_calculate%5Fkey%5Fpoint_Subsystem2_Delay6.fixedpointlog  use_init=off  reset_value=1
  Delay9 : allblocks_alteradspbuilder2/Delay  pipeline=1  pipeline_display=1  ClockPhase=1  use_ena=on  use_sclr=off  allowFloatingPointOverride=on  logOutputs=off  logFile=C:\Users\ASUS\Desktop\sift_fpga_final\Gaussian filter 5x5\tb_dog_test\dog%5Ftest_calculate%5Fkey%5Fpoint_Subsystem2_Delay9.fixedpointlog  use_init=off  reset_value=1
  Memory Delay : allblocks_alteradspbuilder2/Memory Delay  BusType=Unsigned Integer  bwl=8  bwr=0  pipeline=638  pipeline_display=638  ram_type=AUTO  use_ena=on  use_sclr=off  allowFloatingPointOverride=on  logOutputs=off  logFile=C:\Users\ASUS\Desktop\sift_fpga_final\Gaussian filter 5x5\tb_dog_test\dog%5Ftest_calculate%5Fkey%5Fpoint_Subsystem2_Memory+Delay.fixedpointlog
  Memory Delay1 : allblocks_alteradspbuilder2/Memory Delay  BusType=Unsigned Integer  bwl=8  bwr=0  pipeline=638  pipeline_display=638  ram_type=AUTO  use_ena=on  use_sclr=off  allowFloatingPointOverride=on  logOutputs=off  logFile=C:\Users\ASUS\Desktop\sift_fpga_final\Gaussian filter 5x5\tb_dog_test\dog%5Ftest_calculate%5Fkey%5Fpoint_Subsystem2_Memory+Delay1.fixedpointlog
  Out00 : Outport
  Out01 : Outport  Port=2
  Out02 : Outport  Port=3
  Out10 : Outport  Port=4
  Out11 : Outport  Port=5
  Out12 : Outport  Port=6
  Out20 : Outport  Port=7
  Out21 : Outport  Port=8
  Out22 : Outport  Port=9
  wires:
  Delay1/1 -> [data_01], Delay2/1
  Delay/1 -> [data_00], Delay1/1
  Delay9/1 -> [data_21], Delay10/1
  [clken] -> Delay10/2
  [clken] -> Memory Delay1/2
  Delay6/1 -> Memory Delay1/1, [data_12]
  Memory Delay1/1 -> [data_20], Delay9/1
  [clken] -> Delay9/2
  [data_02] -> Out02/1
  [clken] -> Delay1/2
  [clken] -> Delay/2
  [data_in] -> Delay/1
  [clken] -> Delay2/2
  Delay2/1 -> Memory Delay/1, [data_02]
  [data_22] -> Out22/1
  Delay10/1 -> [data_22]
  clken/1 -> [clken]
  [data_21] -> Out21/1
  [data_20] -> Out20/1
  [data_10] -> Out10/1
  Memory Delay/1 -> [data_10], Delay5/1
  [clken] -> Memory Delay/2
  [clken] -> Delay6/2
  Delay5/1 -> [data_11], Delay6/1
  [data_12] -> Out12/1
  [data_00] -> Out00/1
  [data_01] -> Out01/1
  [clken] -> Delay5/2
  [data_11] -> Out11/1
  dataIn/1 -> [data_in]

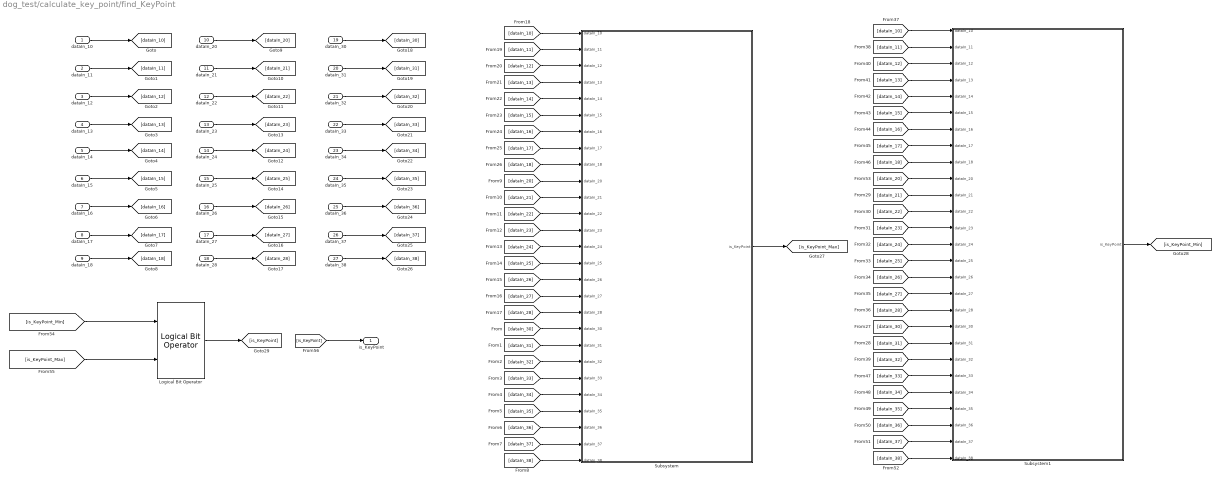
== system dog_test/calculate_key_point/find_KeyPoint ==
  dataIn_10 : Inport
  dataIn_11 : Inport  Port=2
  dataIn_12 : Inport  Port=3
  dataIn_13 : Inport  Port=4
  dataIn_14 : Inport  Port=5
  dataIn_15 : Inport  Port=6
  dataIn_16 : Inport  Port=7
  dataIn_17 : Inport  Port=8
  dataIn_18 : Inport  Port=9
  dataIn_20 : Inport  Port=10
  dataIn_21 : Inport  Port=11
  dataIn_22 : Inport  Port=12
  dataIn_23 : Inport  Port=13
  dataIn_24 : Inport  Port=14
  dataIn_25 : Inport  Port=15
  dataIn_26 : Inport  Port=16
  dataIn_27 : Inport  Port=17
  dataIn_28 : Inport  Port=18
  dataIn_30 : Inport  Port=19
  dataIn_31 : Inport  Port=20
  dataIn_32 : Inport  Port=21
  dataIn_33 : Inport  Port=22
  dataIn_34 : Inport  Port=23
  dataIn_35 : Inport  Port=24
  dataIn_36 : Inport  Port=25
  dataIn_37 : Inport  Port=26
  dataIn_38 : Inport  Port=27
  Logical Bit Operator : allblocks_alteradspbuilder2/Logical Bit Operator  LogicalOperator=OR  user_inputs=2  pipeline_display=0
  Subsystem : Subsystem
  Subsystem1 : Subsystem
  is_KeyPoint : Outport
  wires:
  [dataIn_32] -> Subsystem/21(dataIn_32)
  [dataIn_33] -> Subsystem/22(dataIn_33)
  [dataIn_36] -> Subsystem/25(dataIn_36)
  [dataIn_37] -> Subsystem/26(dataIn_37)
  [dataIn_34] -> Subsystem/23(dataIn_34)
  [dataIn_35] -> Subsystem/24(dataIn_35)
  [dataIn_30] -> Subsystem/19(dataIn_30)
  [dataIn_31] -> Subsystem/20(dataIn_31)
  Subsystem/1(is_KeyPoint) -> [is_KeyPoint_Max]
  [dataIn_28] -> Subsystem/18(dataIn_28)
  [dataIn_26] -> Subsystem/16(dataIn_26)
  [dataIn_22] -> Subsystem/12(dataIn_22)
  [dataIn_27] -> Subsystem/17(dataIn_27)
  [dataIn_20] -> Subsystem/10(dataIn_20)
  [dataIn_23] -> Subsystem/13(dataIn_23)
  [dataIn_24] -> Subsystem/14(dataIn_24)
  [dataIn_21] -> Subsystem/11(dataIn_21)
  [dataIn_25] -> Subsystem/15(dataIn_25)
  [dataIn_10] -> Subsystem/1(dataIn_10)
  [dataIn_11] -> Subsystem/2(dataIn_11)
  [dataIn_12] -> Subsystem/3(dataIn_12)
  dataIn_23/1 -> [dataIn_23]
  dataIn_17/1 -> [dataIn_17]
  dataIn_22/1 -> [dataIn_22]
  dataIn_14/1 -> [dataIn_14]
  dataIn_16/1 -> [dataIn_16]
  dataIn_28/1 -> [dataIn_28]
  dataIn_20/1 -> [dataIn_20]
  dataIn_21/1 -> [dataIn_21]
  dataIn_26/1 -> [dataIn_26]
  dataIn_10/1 -> [dataIn_10]
  dataIn_30/1 -> [dataIn_30]
  dataIn_27/1 -> [dataIn_27]
  dataIn_25/1 -> [dataIn_25]
  dataIn_15/1 -> [dataIn_15]
  dataIn_18/1 -> [dataIn_18]
  dataIn_24/1 -> [dataIn_24]
  dataIn_32/1 -> [dataIn_32]
  dataIn_13/1 -> [dataIn_13]
  dataIn_31/1 -> [dataIn_31]
  [dataIn_14] -> Subsystem/5(dataIn_14)
  dataIn_34/1 -> [dataIn_34]
  dataIn_11/1 -> [dataIn_11]
  [dataIn_17] -> Subsystem/8(dataIn_17)
  dataIn_35/1 -> [dataIn_35]
  dataIn_33/1 -> [dataIn_33]
  dataIn_38/1 -> [dataIn_38]
  [dataIn_13] -> Subsystem/4(dataIn_13)
  [dataIn_16] -> Subsystem/7(dataIn_16)
  [dataIn_15] -> Subsystem/6(dataIn_15)
  dataIn_12/1 -> [dataIn_12]
  [dataIn_18] -> Subsystem/9(dataIn_18)
  dataIn_36/1 -> [dataIn_36]
  dataIn_37/1 -> [dataIn_37]
  [dataIn_38] -> Subsystem/27(dataIn_38)
  Subsystem1/1(is_KeyPoint) -> [is_KeyPoint_Min]
  [dataIn_11] -> Subsystem1/2(dataIn_11)
  [dataIn_12] -> Subsystem1/3(dataIn_12)
  [dataIn_13] -> Subsystem1/4(dataIn_13)
  [dataIn_15] -> Subsystem1/6(dataIn_15)
  [dataIn_16] -> Subsystem1/7(dataIn_16)
  [dataIn_17] -> Subsystem1/8(dataIn_17)
  [dataIn_18] -> Subsystem1/9(dataIn_18)
  [dataIn_31] -> Subsystem1/20(dataIn_31)
  [dataIn_14] -> Subsystem1/5(dataIn_14)
  [is_KeyPoint] -> is_KeyPoint/1
  [dataIn_33] -> Subsystem1/22(dataIn_33)
  [dataIn_32] -> Subsystem1/21(dataIn_32)
  [dataIn_34] -> Subsystem1/23(dataIn_34)
  [dataIn_35] -> Subsystem1/24(dataIn_35)
  [dataIn_36] -> Subsystem1/25(dataIn_36)
  [dataIn_21] -> Subsystem1/11(dataIn_21)
  [dataIn_22] -> Subsystem1/12(dataIn_22)
  [dataIn_23] -> Subsystem1/13(dataIn_23)
  [dataIn_25] -> Subsystem1/15(dataIn_25)
  [dataIn_24] -> Subsystem1/14(dataIn_24)
  [dataIn_38] -> Subsystem1/27(dataIn_38)
  [dataIn_20] -> Subsystem1/10(dataIn_20)
  [dataIn_26] -> Subsystem1/16(dataIn_26)
  [dataIn_30] -> Subsystem1/19(dataIn_30)
  [dataIn_27] -> Subsystem1/17(dataIn_27)
  [dataIn_37] -> Subsystem1/26(dataIn_37)
  [dataIn_28] -> Subsystem1/18(dataIn_28)
  [dataIn_10] -> Subsystem1/1(dataIn_10)
  Logical Bit Operator/1 -> [is_KeyPoint]
  [is_KeyPoint_Min] -> Logical Bit Operator/1
  [is_KeyPoint_Max] -> Logical Bit Operator/2
